simulink model "TwoMassSystem"  (R2014a)
settings: Solver=ode45  StartTime=0.0  StopTime=t_end  FixedStep=dt  MaxStep=dt  RelTol=1e-3
values from neighbouring files (symbols this model uses):
  K1 = Element_Spring(1)    [OneMassOneSpring.m]
  K2 = 0    [OneMassOneSpring.m]
  M1 = Node_Mass(2)    [OneMassOneSpring.m]
settings Model: Creator=cloughj  LastModifiedBy=cloughj

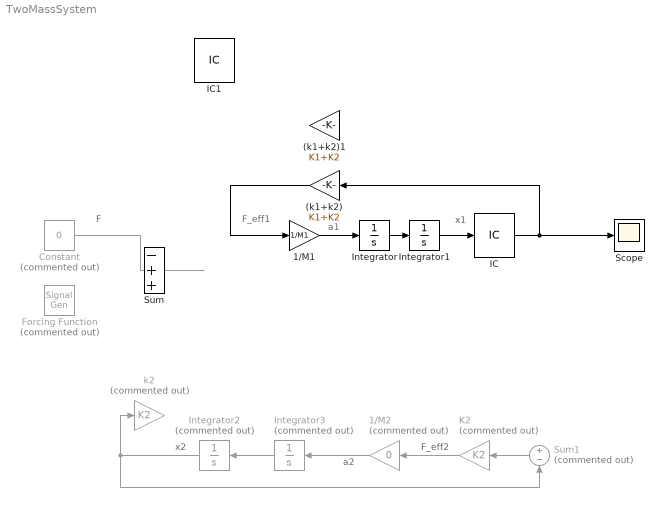
== system TwoMassSystem ==
  note: F_eff2
  note: a2
  note: x2
  note: x1
  note: a1
  note: F_eff1
  note: F
  (k1+k2) : Gain  Gain=K1+K2
  (k1+k2)1 : Gain  Gain=K1+K2
  1/M1 : Gain  Gain=1/M1
  1/M2 : Gain  Commented=on  Gain=0
  Constant : Constant  Commented=on  Value=0
  Forcing Function : SignalGenerator  Commented=on  WaveForm=square
  IC : InitialCondition
  IC1 : InitialCondition
  Integrator : Integrator
  Integrator1 : Integrator
  Integrator2 : Integrator  Commented=on
  Integrator3 : Integrator  Commented=on
  K2 : Gain  Commented=on  Gain=K2
  Scope : Scope
      settings: YMin=-1.5e-24  YMax=8e-24  SaveName=TwoMassPositions
  Sum : Sum  Inputs=-++
  Sum1 : Sum  Commented=on  Inputs=+-
  k2 : Gain  Commented=on  Gain=K2
  wires:
  Constant/1 -> ?
  IC/1 -> Scope/1, (k1+k2)/1
  Integrator2/1 -> Sum1/2, k2/1
  Integrator3/1 -> Integrator2/1
  1/M2/1 -> Integrator3/1
  K2/1 -> 1/M2/1
  Sum1/1 -> K2/1
  (k1+k2)/1 -> 1/M1/1
  Integrator/1 -> Integrator1/1
  1/M1/1 -> Integrator/1
  Integrator1/1 -> IC/1
